simulink model "lab1"  (R2021b)
settings: Solver=VariableStepAuto  StartTime=0.0  StopTime=20.0  RelTol=1e-3
settings Model: Creator=user  LastModifiedBy=user

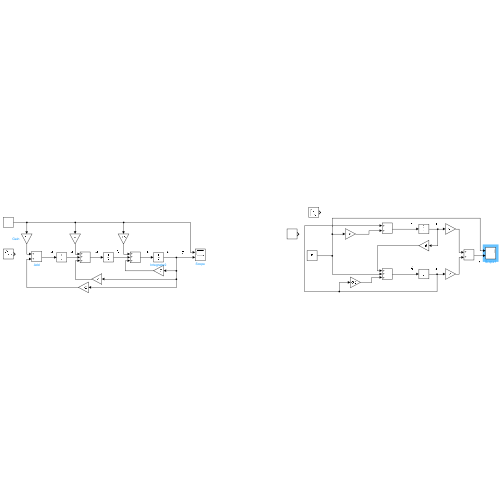
[thumbnail: Simulink's stored preview of the top-level diagram]
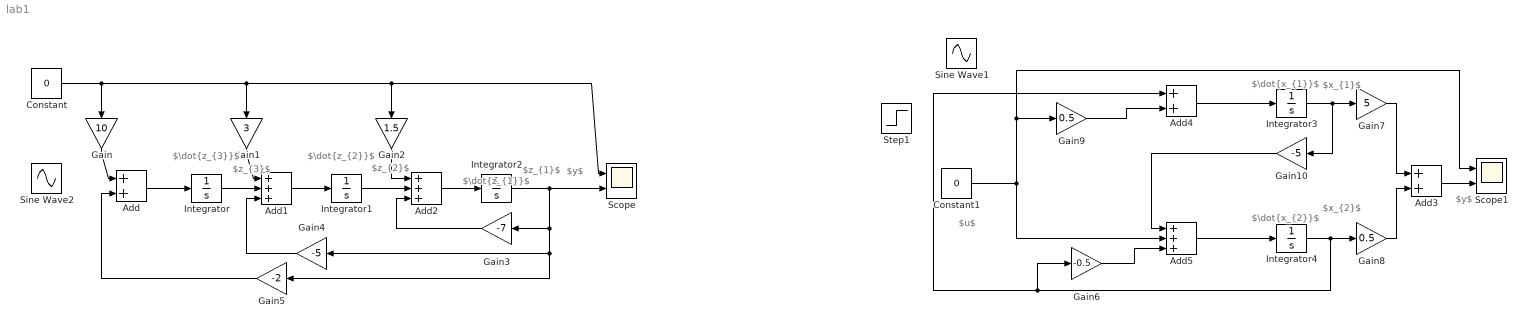
== system lab1 ==
  note: $y$
  note: $u$
  note: $y$
  note: $\dot{z_{1}}$
  note: $z_{1}$
  note: $z_{2}$
  note: $z_{3}$
  note: $\dot{z_{2}}$
  note: $\dot{z_{3}}$
  note: $x_{1}$
  note: $\dot{x_{1}}$
  note: $x_{2}$
  note: $\dot{x_{2}}$
  Add : Sum
  Add1 : Sum  Inputs=+++
  Add2 : Sum  Inputs=+++
  Add3 : Sum
  Add4 : Sum
  Add5 : Sum  Inputs=+++
  Constant : Constant  Value=0
  Constant1 : Constant  Value=0
  Gain : Gain  Gain=10
  Gain1 : Gain  Gain=3
  Gain10 : Gain  Gain=-5
  Gain2 : Gain  Gain=1.5
  Gain3 : Gain  Gain=-7
  Gain4 : Gain  Gain=-5
  Gain5 : Gain  Gain=-2
  Gain6 : Gain  Gain=-0.5
  Gain7 : Gain  Gain=5
  Gain8 : Gain  Gain=0.5
  Gain9 : Gain  Gain=0.5
  Integrator : Integrator  InitialCondition=-8.5
  Integrator1 : Integrator  InitialCondition=6.5
  Integrator2 : Integrator  InitialCondition=1
  Integrator3 : Integrator  InitialCondition=0.2
  Integrator4 : Integrator  InitialCondition=-0.1
  Scope : Scope  NumInputPorts=2
  Scope1 : Scope  NumInputPorts=2
  Sine Wave1 : Sin  Amplitude=2  SampleTime=0
  Sine Wave2 : Sin  Amplitude=2  SampleTime=0
  Step1 : Step  SampleTime=0
  wires:
  Constant/1 -> Scope/1, Gain2/1, Gain1/1, Gain/1
  Integrator2/1 -> Scope/2, Gain5/1, Gain4/1, Gain3/1
  Gain/1 -> Add/1
  Gain5/1 -> Add/2
  Add/1 -> Integrator/1
  Integrator/1 -> Add1/2
  Add1/1 -> Integrator1/1
  Integrator1/1 -> Add2/2
  Add2/1 -> Integrator2/1
  Gain1/1 -> Add1/1
  Gain2/1 -> Add2/1
  Gain3/1 -> Add2/3
  Gain4/1 -> Add1/3
  Integrator3/1 -> Gain10/1, Gain7/1
  Integrator4/1 -> Add4/1, Gain6/1, Gain8/1
  Gain8/1 -> Add3/2
  Gain7/1 -> Add3/1
  Add3/1 -> Scope1/2
  Constant1/1 -> Scope1/1, Gain9/1, Add5/2
  Gain9/1 -> Add4/2
  Add4/1 -> Integrator3/1
  Add5/1 -> Integrator4/1
  Gain10/1 -> Add5/1
  Gain6/1 -> Add5/3
